simulink model "controlador_integrador_LPV_real"  (R2018b)
settings: Solver=FixedStepAuto  StartTime=0.0  StopTime=timeout  FixedStep=T  RelTol=1e-3
values from neighbouring files (symbols this model uses):
  K1_ = K1_lmi(1:2)    [data_2_real.m]
  K2_ = K2_lmi(1:2)    [data_2_real.m]
  Ka_ = [K1_lmi(3) K2_lmi(3)]    [data_2_real.m]
  rho = max(u_s)    [data_2_real.m]
  T = 5.2632    [data_2_real.m]
settings Model: Creator=tarsis  LastModifiedBy=tarsis

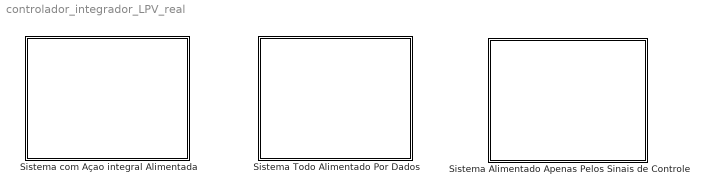
== system controlador_integrador_LPV_real ==
  Sistema Alimentado Apenas Pelos Sinais de Controle : Subsystem
  Sistema Todo Alimentado Por Dados : Subsystem
  Sistema com Açao integral Alimentada : Subsystem

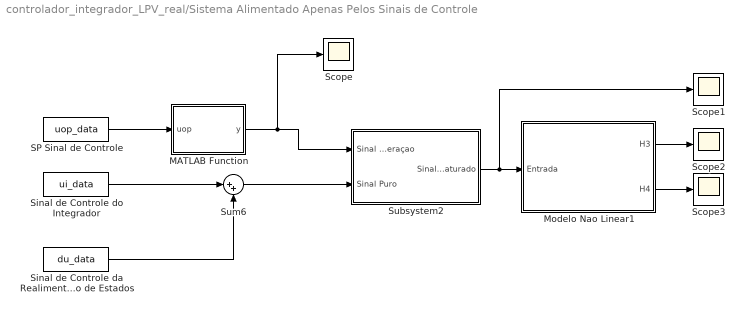
== system controlador_integrador_LPV_real/Sistema Alimentado Apenas Pelos Sinais de Controle ==
  MATLAB Function : MATLAB Function  TreatAsAtomicUnit=on
  Modelo Nao Linear1 : Subsystem
  SP Sinal de Controle : FromWorkspace  VariableName=uop_data  SampleTime=T  Interpolate=off  OutputAfterFinalValue=Setting to zero
  Scope{,1..3} (4 alike) : Scope
  Sinal de Controle da Realimentaçao de Estados : FromWorkspace  VariableName=du_data  SampleTime=T  Interpolate=off  OutputAfterFinalValue=Setting to zero
  Sinal de Controle do Integrador : FromWorkspace  VariableName=ui_data  SampleTime=T  Interpolate=off  OutputAfterFinalValue=Setting to zero
  Subsystem2 : Subsystem
  Sum6 : Sum  Inputs=|++
  wires:
  Sum6/1 -> Subsystem2/2(Sinal Puro)
  Modelo Nao Linear1/2(H4) -> Scope3/1
  Sinal de Controle do Integrador/1 -> Sum6/1
  Subsystem2/1(Sinal Saturado) -> Modelo Nao Linear1/1(Entrada), Scope1/1
  Sinal de Controle da Realimentaçao de Estados/1 -> Sum6/2
  Modelo Nao Linear1/1(H3) -> Scope2/1
  SP Sinal de Controle/1 -> MATLAB Function/1(uop)
  MATLAB Function/1(y) -> Scope/1, Subsystem2/1(Sinal de Operaçao)

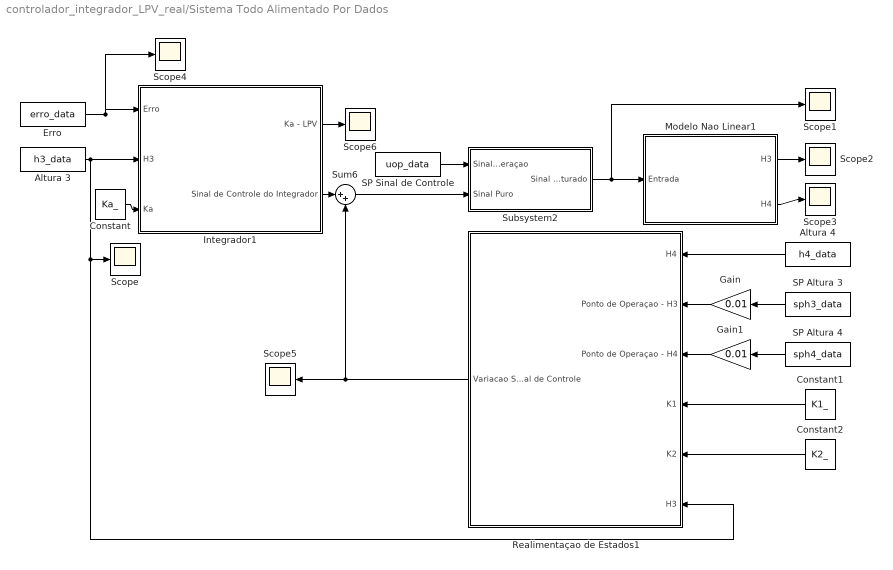
== system controlador_integrador_LPV_real/Sistema Todo Alimentado Por Dados ==
  Altura 3 : FromWorkspace  VariableName=h3_data  SampleTime=T  Interpolate=off  OutputAfterFinalValue=Setting to zero
  Altura 4 : FromWorkspace  VariableName=h4_data  SampleTime=T  Interpolate=off  OutputAfterFinalValue=Setting to zero
  Constant : Constant  Value=Ka_  VectorParams1D=off
  Constant1 : Constant  Value=K1_  VectorParams1D=off
  Constant2 : Constant  Value=K2_  VectorParams1D=off
  Erro : FromWorkspace  VariableName=erro_data  SampleTime=T  Interpolate=off  OutputAfterFinalValue=Setting to zero
  Gain : Gain  Gain=0.01
  Gain1 : Gain  Gain=0.01
  Integrador1 : Subsystem
  Modelo Nao Linear1 : Subsystem
  Realimentaçao de Estados1 : Subsystem
  SP Altura 3 : FromWorkspace  VariableName=sph3_data  SampleTime=T  Interpolate=off  OutputAfterFinalValue=Setting to zero
  SP Altura 4 : FromWorkspace  VariableName=sph4_data  SampleTime=T  Interpolate=off  OutputAfterFinalValue=Setting to zero
  SP Sinal de Controle : FromWorkspace  VariableName=uop_data  SampleTime=T  Interpolate=off  OutputAfterFinalValue=Setting to zero
  Scope{,1..6} (7 alike) : Scope
  Subsystem2 : Subsystem
  Sum6 : Sum  Inputs=|++
  wires:
  Modelo Nao Linear1/1(H3) -> Scope2/1
  Constant2/1 -> Realimentaçao de Estados1/5(K2)
  Gain1/1 -> Realimentaçao de Estados1/3(Ponto de Operaçao - H4)
  Erro/1 -> Scope4/1, Integrador1/1(Erro)
  Sum6/1 -> Subsystem2/2(Sinal Puro)
  SP Altura 3/1 -> Gain/1
  Altura 3/1 -> Realimentaçao de Estados1/6(H3), Scope/1, Integrador1/2(H3)
  SP Altura 4/1 -> Gain1/1
  Altura 4/1 -> Realimentaçao de Estados1/1(H4)
  Modelo Nao Linear1/2(H4) -> Scope3/1
  Integrador1/2(Sinal de Controle do Integrador) -> Sum6/1
  Integrador1/1(Ka - LPV) -> Scope6/1
  SP Sinal de Controle/1 -> Subsystem2/1(Sinal de Operaçao)
  Constant1/1 -> Realimentaçao de Estados1/4(K1)
  Realimentaçao de Estados1/1(Variacao Sinal de Controle) -> Scope5/1, Sum6/2
  Gain/1 -> Realimentaçao de Estados1/2(Ponto de Operaçao - H3)
  Subsystem2/1(Sinal Saturado) -> Scope1/1, Modelo Nao Linear1/1(Entrada)
  Constant/1 -> Integrador1/3(Ka)

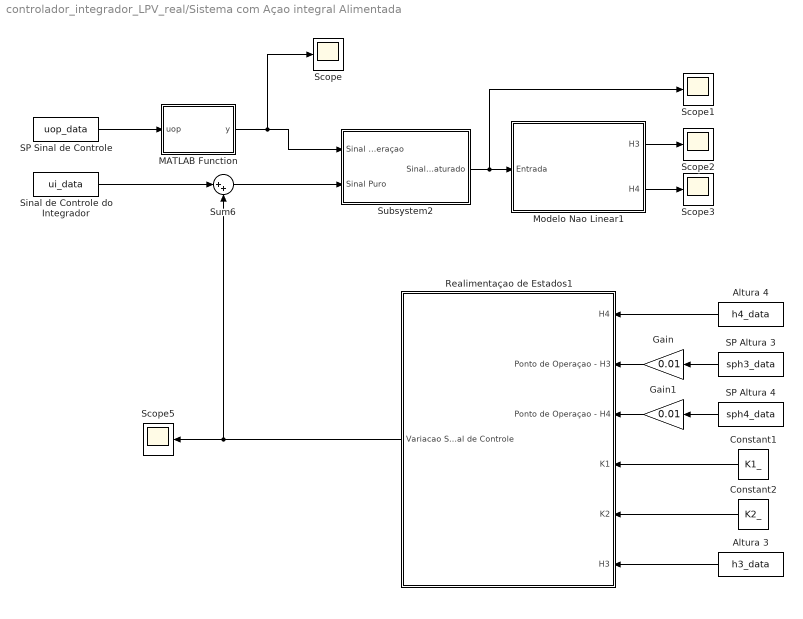
== system controlador_integrador_LPV_real/Sistema com Açao integral Alimentada ==
  Altura 3 : FromWorkspace  VariableName=h3_data  SampleTime=T  Interpolate=off  OutputAfterFinalValue=Setting to zero
  Altura 4 : FromWorkspace  VariableName=h4_data  SampleTime=T  Interpolate=off  OutputAfterFinalValue=Setting to zero
  Constant1 : Constant  Value=K1_  VectorParams1D=off
  Constant2 : Constant  Value=K2_  VectorParams1D=off
  Gain : Gain  Gain=0.01
  Gain1 : Gain  Gain=0.01
  MATLAB Function : MATLAB Function  TreatAsAtomicUnit=on
  Modelo Nao Linear1 : Subsystem
  Realimentaçao de Estados1 : Subsystem
  SP Altura 3 : FromWorkspace  VariableName=sph3_data  SampleTime=T  Interpolate=off  OutputAfterFinalValue=Setting to zero
  SP Altura 4 : FromWorkspace  VariableName=sph4_data  SampleTime=T  Interpolate=off  OutputAfterFinalValue=Setting to zero
  SP Sinal de Controle : FromWorkspace  VariableName=uop_data  SampleTime=T  Interpolate=off  OutputAfterFinalValue=Setting to zero
  Scope{,1..3,5} (5 alike) : Scope
  Sinal de Controle do Integrador : FromWorkspace  VariableName=ui_data  SampleTime=T  Interpolate=off  OutputAfterFinalValue=Setting to zero
  Subsystem2 : Subsystem
  Sum6 : Sum  Inputs=|++
  wires:
  Modelo Nao Linear1/1(H3) -> Scope2/1
  Sum6/1 -> Subsystem2/2(Sinal Puro)
  Subsystem2/1(Sinal Saturado) -> Modelo Nao Linear1/1(Entrada), Scope1/1
  Modelo Nao Linear1/2(H4) -> Scope3/1
  MATLAB Function/1(y) -> Scope/1, Subsystem2/1(Sinal de Operaçao)
  SP Sinal de Controle/1 -> MATLAB Function/1(uop)
  Sinal de Controle do Integrador/1 -> Sum6/1
  Constant1/1 -> Realimentaçao de Estados1/4(K1)
  Gain/1 -> Realimentaçao de Estados1/2(Ponto de Operaçao - H3)
  Altura 4/1 -> Realimentaçao de Estados1/1(H4)
  Gain1/1 -> Realimentaçao de Estados1/3(Ponto de Operaçao - H4)
  Constant2/1 -> Realimentaçao de Estados1/5(K2)
  Realimentaçao de Estados1/1(Variacao Sinal de Controle) -> Sum6/2, Scope5/1
  SP Altura 4/1 -> Gain1/1
  SP Altura 3/1 -> Gain/1
  Altura 3/1 -> Realimentaçao de Estados1/6(H3)

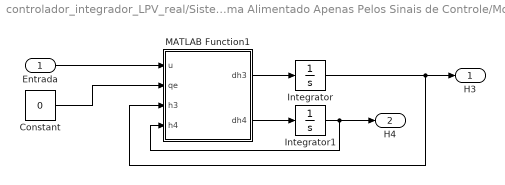
== system controlador_integrador_LPV_real/Sistema Alimentado Apenas Pelos Sinais de Controle/Modelo Nao Linear1 ==
  Entrada : Inport
  Constant : Constant  Value=0
  Integrator : Integrator
  Integrator1 : Integrator
  MATLAB Function1 : MATLAB Function  TreatAsAtomicUnit=on  SystemSampleTime=T
  H3 : Outport
  H4 : Outport  Port=2
  wires:
  Integrator1/1 -> H4/1, MATLAB Function1/4(h4)
  Entrada/1 -> MATLAB Function1/1(u)
  MATLAB Function1/2(dh4) -> Integrator1/1
  Integrator/1 -> H3/1, MATLAB Function1/3(h3)
  MATLAB Function1/1(dh3) -> Integrator/1
  Constant/1 -> MATLAB Function1/2(qe)

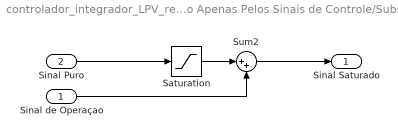
== system controlador_integrador_LPV_real/Sistema Alimentado Apenas Pelos Sinais de Controle/Subsystem2 ==
  Sinal de Operaçao : Inport
  Sinal Puro : Inport  Port=2
  Saturation : Saturate  UpperLimit=rho  LowerLimit=-rho
  Sum2 : Sum  Inputs=|++
  Sinal Saturado : Outport
  wires:
  Saturation/1 -> Sum2/1
  Sinal de Operaçao/1 -> Sum2/2
  Sum2/1 -> Sinal Saturado/1
  Sinal Puro/1 -> Saturation/1

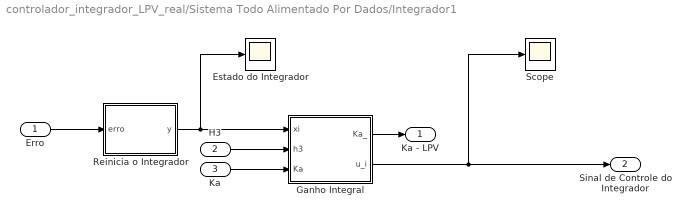
== system controlador_integrador_LPV_real/Sistema Todo Alimentado Por Dados/Integrador1 ==
  Erro : Inport
  H3 : Inport  Port=2
  Ka : Inport  Port=3
  Estado do Integrador : Scope
  Ganho Integral : MATLAB Function  TreatAsAtomicUnit=on
  Reinicia o Integrador : MATLAB Function  TreatAsAtomicUnit=on  SystemSampleTime=T
  Scope : Scope
  Ka - LPV : Outport
  Sinal de Controle do Integrador : Outport  Port=2
  wires:
  H3/1 -> Ganho Integral/2(h3)
  Reinicia o Integrador/1(y) -> Estado do Integrador/1, Ganho Integral/1(xi)
  Ganho Integral/2(u_i) -> Sinal de Controle do Integrador/1, Scope/1
  Erro/1 -> Reinicia o Integrador/1(erro)
  Ka/1 -> Ganho Integral/3(Ka)
  Ganho Integral/1(Ka_) -> Ka - LPV/1

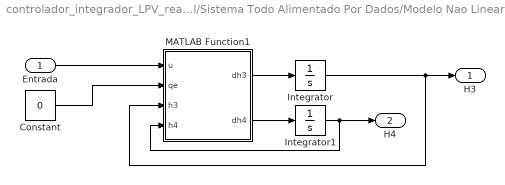
== system controlador_integrador_LPV_real/Sistema Todo Alimentado Por Dados/Modelo Nao Linear1 ==
  Entrada : Inport
  Constant : Constant  Value=0
  Integrator : Integrator
  Integrator1 : Integrator
  MATLAB Function1 : MATLAB Function  TreatAsAtomicUnit=on  SystemSampleTime=T
  H3 : Outport
  H4 : Outport  Port=2
  wires:
  Integrator1/1 -> H4/1, MATLAB Function1/4(h4)
  Entrada/1 -> MATLAB Function1/1(u)
  MATLAB Function1/2(dh4) -> Integrator1/1
  Integrator/1 -> H3/1, MATLAB Function1/3(h3)
  MATLAB Function1/1(dh3) -> Integrator/1
  Constant/1 -> MATLAB Function1/2(qe)

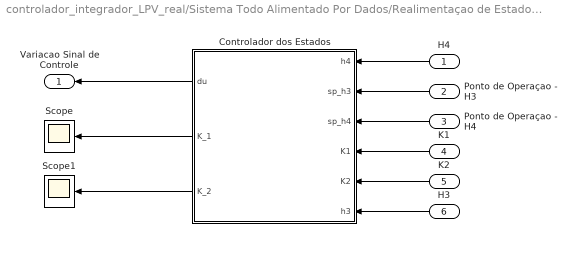
== system controlador_integrador_LPV_real/Sistema Todo Alimentado Por Dados/Realimentaçao de Estados1 ==
  H4 : Inport
  Ponto de Operaçao - H3 : Inport  Port=2
  Ponto de Operaçao - H4 : Inport  Port=3
  K1 : Inport  Port=4
  K2 : Inport  Port=5
  H3 : Inport  Port=6
  Controlador dos Estados : MATLAB Function  TreatAsAtomicUnit=on  SystemSampleTime=T
  Scope : Scope
  Scope1 : Scope
  Variacao Sinal de Controle : Outport
  wires:
  H4/1 -> Controlador dos Estados/1(h4)
  H3/1 -> Controlador dos Estados/6(h3)
  Controlador dos Estados/1(du) -> Variacao Sinal de Controle/1
  Ponto de Operaçao - H3/1 -> Controlador dos Estados/2(sp_h3)
  Ponto de Operaçao - H4/1 -> Controlador dos Estados/3(sp_h4)
  K1/1 -> Controlador dos Estados/4(K1)
  K2/1 -> Controlador dos Estados/5(K2)
  Controlador dos Estados/2(K_1) -> Scope/1
  Controlador dos Estados/3(K_2) -> Scope1/1

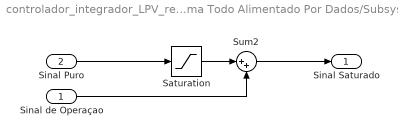
== system controlador_integrador_LPV_real/Sistema Todo Alimentado Por Dados/Subsystem2 ==
  Sinal de Operaçao : Inport
  Sinal Puro : Inport  Port=2
  Saturation : Saturate  UpperLimit=rho  LowerLimit=-rho
  Sum2 : Sum  Inputs=|++
  Sinal Saturado : Outport
  wires:
  Saturation/1 -> Sum2/1
  Sinal de Operaçao/1 -> Sum2/2
  Sum2/1 -> Sinal Saturado/1
  Sinal Puro/1 -> Saturation/1

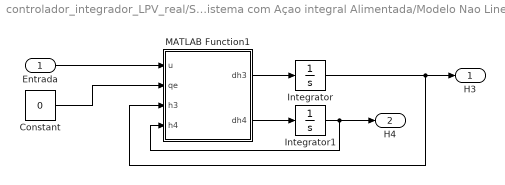
== system controlador_integrador_LPV_real/Sistema com Açao integral Alimentada/Modelo Nao Linear1 ==
  Entrada : Inport
  Constant : Constant  Value=0
  Integrator : Integrator
  Integrator1 : Integrator
  MATLAB Function1 : MATLAB Function  TreatAsAtomicUnit=on  SystemSampleTime=T
  H3 : Outport
  H4 : Outport  Port=2
  wires:
  Integrator1/1 -> H4/1, MATLAB Function1/4(h4)
  Entrada/1 -> MATLAB Function1/1(u)
  MATLAB Function1/2(dh4) -> Integrator1/1
  Integrator/1 -> H3/1, MATLAB Function1/3(h3)
  MATLAB Function1/1(dh3) -> Integrator/1
  Constant/1 -> MATLAB Function1/2(qe)

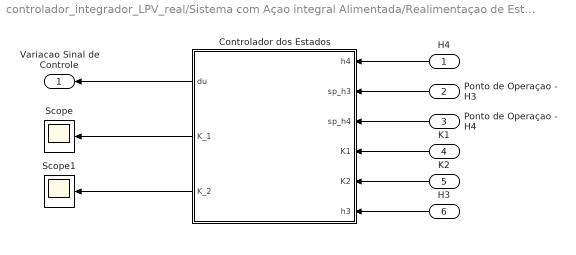
== system controlador_integrador_LPV_real/Sistema com Açao integral Alimentada/Realimentaçao de Estados1 ==
  H4 : Inport
  Ponto de Operaçao - H3 : Inport  Port=2
  Ponto de Operaçao - H4 : Inport  Port=3
  K1 : Inport  Port=4
  K2 : Inport  Port=5
  H3 : Inport  Port=6
  Controlador dos Estados : MATLAB Function  TreatAsAtomicUnit=on  SystemSampleTime=T
  Scope : Scope
  Scope1 : Scope
  Variacao Sinal de Controle : Outport
  wires:
  H4/1 -> Controlador dos Estados/1(h4)
  H3/1 -> Controlador dos Estados/6(h3)
  Controlador dos Estados/1(du) -> Variacao Sinal de Controle/1
  Ponto de Operaçao - H3/1 -> Controlador dos Estados/2(sp_h3)
  Ponto de Operaçao - H4/1 -> Controlador dos Estados/3(sp_h4)
  K1/1 -> Controlador dos Estados/4(K1)
  K2/1 -> Controlador dos Estados/5(K2)
  Controlador dos Estados/2(K_1) -> Scope/1
  Controlador dos Estados/3(K_2) -> Scope1/1

== system controlador_integrador_LPV_real/Sistema com Açao integral Alimentada/Subsystem2 ==
  Sinal de Operaçao : Inport
  Sinal Puro : Inport  Port=2
  Saturation : Saturate  UpperLimit=rho  LowerLimit=-rho
  Sum2 : Sum  Inputs=|++
  Sinal Saturado : Outport
  wires:
  Saturation/1 -> Sum2/1
  Sinal de Operaçao/1 -> Sum2/2
  Sum2/1 -> Sinal Saturado/1
  Sinal Puro/1 -> Saturation/1

== matlab function controlador_integrador_LPV_real/Sistema com Açao integral Alimentada/MATLAB Function ==
  data: uop input; y output
function y = fcn(uop)
if uop == 0
    y = 50;
else
    y = uop;
end

== matlab function controlador_integrador_LPV_real/Sistema Alimentado Apenas Pelos Sinais de Controle/MATLAB Function ==
  data: uop input; y output
function y = fcn(uop)
if uop == 0
    y = 50;
else
    y = uop;
end

== matlab function controlador_integrador_LPV_real/Sistema Alimentado Apenas Pelos Sinais de Controle/Modelo Nao Linear1/MATLAB Function1 ==
  data: u input; qe input; dh3 output; h3 input; h4 input; dh4 output
function [dh3,dh4] = fcn(u,qe,h3,h4)
qi = (16.4*u + 357.3)*1e-6;
q12 = 33.51e-4*(h4 - h3) + 43.12e-5;
qout = (87.07e-5*sqrt(h3) + 30.99e-5);
A1 = (pi*(31)^2)*1e-4;
A2 = - 0.88629272879272778105782609278436*h3^16 + 6.0267905557905489111932174309337*h3^15 - 20.80464391736738395516887057851*h3^14 + 47.68494439008527766774004035511*h3^13 - 82.573907447205791291786792565001*h3^12 + 116.28257881925208875326233578017*h3^11 - 139.30893428077013388311346843447*h3^10 + 144.80767028205944702410747888441*h3^9 - 129.2475129476872169884635810807*h3^8 + 96.099152680911332924853135955618*h3^7 - 55.593870964701796673125553833866*h3^6 + 21.451550218200266654046211819752*h3^5 - 5.9275208717979510465216954484015*h3^4 + 3.9856416105248966168880953176109*h3^3 - 2.0902185091906828919771687989635*h3^2 - 0.061481774188906647716430580264178*h3 + 0.32722421068834535751546101783638;
dh4 = (qi - q12)/A1;
dh3 = (q12 - qout + qe)/A2;

== matlab function controlador_integrador_LPV_real/Sistema com Açao integral Alimentada/Modelo Nao Linear1/MATLAB Function1 ==
  data: u input; qe input; dh3 output; h3 input; h4 input; dh4 output
function [dh3,dh4] = fcn(u,qe,h3,h4)
qi = (16.4*u + 357.3)*1e-6;
q12 = 33.51e-4*(h4 - h3) + 43.12e-5;
qout = (87.07e-5*sqrt(h3) + 30.99e-5);
A1 = (pi*(31)^2)*1e-4;
A2 = - 0.88629272879272778105782609278436*h3^16 + 6.0267905557905489111932174309337*h3^15 - 20.80464391736738395516887057851*h3^14 + 47.68494439008527766774004035511*h3^13 - 82.573907447205791291786792565001*h3^12 + 116.28257881925208875326233578017*h3^11 - 139.30893428077013388311346843447*h3^10 + 144.80767028205944702410747888441*h3^9 - 129.2475129476872169884635810807*h3^8 + 96.099152680911332924853135955618*h3^7 - 55.593870964701796673125553833866*h3^6 + 21.451550218200266654046211819752*h3^5 - 5.9275208717979510465216954484015*h3^4 + 3.9856416105248966168880953176109*h3^3 - 2.0902185091906828919771687989635*h3^2 - 0.061481774188906647716430580264178*h3 + 0.32722421068834535751546101783638;
dh4 = (qi - q12)/A1;
dh3 = (q12 - qout + qe)/A2;

== matlab function controlador_integrador_LPV_real/Sistema com Açao integral Alimentada/Realimentaçao de Estados1/Controlador dos Estados ==
  data: h4 input; sp_h3 input; sp_h4 input; K1 input; K2 input; h3 input; du output; K_1 output; K_2 output
function [du,K_1,K_2]  = fcn(h4,sp_h3,sp_h4,K1,K2,h3)
% Saída do Modelo não Linear
h = [h4 h3]';
% Pontos de Operação
sp_h = [sp_h4 sp_h3]';
% Equação do Ganho LPV em função de alfa
K = h3*0.05*(K2 - K1) + 2.4*K1 - 1.4*K2;
% Separando os valores de K
K_1 = K(1);
K_2 = K(2);
% Realimentação do Estados
du = K*(h - sp_h);

== matlab function controlador_integrador_LPV_real/Sistema Todo Alimentado Por Dados/Modelo Nao Linear1/MATLAB Function1 ==
  data: u input; qe input; dh3 output; h3 input; h4 input; dh4 output
function [dh3,dh4] = fcn(u,qe,h3,h4)
qi = (16.4*u + 357.3)*1e-6;
q12 = 33.51e-4*(h4 - h3) + 43.12e-5;
qout = (87.07e-5*sqrt(h3) + 30.99e-5);
A1 = (pi*(31)^2)*1e-4;
A2 = - 0.88629272879272778105782609278436*h3^16 + 6.0267905557905489111932174309337*h3^15 - 20.80464391736738395516887057851*h3^14 + 47.68494439008527766774004035511*h3^13 - 82.573907447205791291786792565001*h3^12 + 116.28257881925208875326233578017*h3^11 - 139.30893428077013388311346843447*h3^10 + 144.80767028205944702410747888441*h3^9 - 129.2475129476872169884635810807*h3^8 + 96.099152680911332924853135955618*h3^7 - 55.593870964701796673125553833866*h3^6 + 21.451550218200266654046211819752*h3^5 - 5.9275208717979510465216954484015*h3^4 + 3.9856416105248966168880953176109*h3^3 - 2.0902185091906828919771687989635*h3^2 - 0.061481774188906647716430580264178*h3 + 0.32722421068834535751546101783638;
dh4 = (qi - q12)/A1;
dh3 = (q12 - qout + qe)/A2;

== matlab function controlador_integrador_LPV_real/Sistema Todo Alimentado Por Dados/Realimentaçao de Estados1/Controlador dos Estados ==
  data: h4 input; sp_h3 input; sp_h4 input; K1 input; K2 input; h3 input; du output; K_1 output; K_2 output
function [du,K_1,K_2]  = fcn(h4,sp_h3,sp_h4,K1,K2,h3)
% Saída do Modelo não Linear
h = [h4 h3]';
% Pontos de Operação
sp_h = [sp_h4 sp_h3]';
% Equação do Ganho LPV em função de alfa
K = h3*0.05*(K2 - K1) + 2.4*K1 - 1.4*K2;
% Separando os valores de K
K_1 = K(1);
K_2 = K(2);
% Realimentação do Estados
du = K*(h - sp_h);

== matlab function controlador_integrador_LPV_real/Sistema Todo Alimentado Por Dados/Integrador1/Ganho Integral ==
  data: Ka_ output; xi input; u_i output; h3 input; Ka input
function [Ka_,u_i] = fcn(xi,h3,Ka)

Ka_ = h3*0.05*(Ka(2) - Ka(1)) + 2.4*Ka(1) - 1.4*Ka(2);
u_i = xi*Ka_;

== matlab function controlador_integrador_LPV_real/Sistema Todo Alimentado Por Dados/Integrador1/Reinicia o Integrador ==
  settings: updateMethod=DISCRETE
  data: erro input; y output
function y = fcn(erro)
% Estado do integrador
persistent xi
if isempty(xi)
    xi = 0;
end
% Ação integral
xi = erro + xi;
y = xi;
